simulink model "Simple_4Quad_payload_05"  (R2018b)
settings: Solver=VariableStepAuto  StartTime=0.0  StopTime=60  RelTol=1e-3
InitFcn:
  | Simple_4Quad_payload_05_const
values from neighbouring files (symbols this model uses):
  All_rho = [d1 0 0 ... (first row only)    [Colab_4Quad_model_01_const.m]    (also in Colab_4Quad_model_02_const.m; Simple_4Quad_payload_04_const.m; Simple_4Quad_payload_05_const.m; Simple_4Quad_payload_06_const.m)
  B_ob = [zeros(3);eye(3)]    [Simple_4Quad_payload_04_const.m]    (also in Simple_4Quad_payload_05_const.m; Simple_4Quad_payload_06_const.m; Simple_4Quad_payload_07_const.m; Simple_4Quad_payload_08_const.m)
  BBT_inv = ((B'*B)^(-1))*B'    [Simple_2Quad_payload_03_const.m]    (also in Simple_4Quad_payload_04_const.m = ((BR'*BR)^(-1))*BR'; Simple_4Quad_payload_05_const.m = ((BR'*BR)^(-1))*BR'; Simple_4Quad_payload_06_const.m = ((BR'*BR)^(-1))*BR'; Simple_4Quad_payload_07_const.m = ((BR'*BR)^(-1))*BR')
  BR = 1e0*eye(n)    [Simple_4Quad_payload_04_const.m]    (also in Simple_4Quad_payload_05_const.m; Simple_4Quad_payload_06_const.m; Simple_4Quad_payload_07_const.m; Simple_4Quad_payload_08_const.m)
  C_ob = [eye(3) zeros(3)]    [Simple_4Quad_payload_04_const.m]    (also in Simple_4Quad_payload_05_const.m; Simple_4Quad_payload_06_const.m; Simple_4Quad_payload_07_const.m; Simple_4Quad_payload_08_const.m)
  d1 = 0.25    [Colab_4Quad_model_01_const.m]    (also in Colab_4Quad_model_02_const.m = 0.5; Simple_4Quad_payload_01_const.m = 1; Simple_4Quad_payload_02_const.m = 1; Simple_4Quad_payload_03_const.m = 1)
  d2 = 0.25    [Colab_4Quad_model_01_const.m]    (also in Colab_4Quad_model_02_const.m = 0.5; Simple_4Quad_payload_01_const.m = 1; Simple_4Quad_payload_02_const.m = 1; Simple_4Quad_payload_03_const.m = 1)
  Des_rel_dist = 2    [Simple_4Quad_payload_01_const.m]    (also in Simple_4Quad_payload_02_const.m = 4; Simple_4Quad_payload_03_const.m = 4; Simple_4Quad_payload_04_const.m; Simple_4Quad_payload_05_const.m)
  g = 9.81    [Colab_4Quad_model_01_const.m]    (also in Colab_4Quad_model_02_const.m; Simple_2Quad_payload_01_const.m; Simple_2Quad_payload_02_const.m; Simple_2Quad_payload_03_const.m)
  gamma_0 = 1e-0*diag([1e-3;1e-0])    [Simple_2Quad_payload_03_const.m]    (also in Simple_4Quad_payload_04_const.m = 1e-0*diag([1e-6*ones(3,1);1e-0*ones(3,1)]); Simple_4Quad_payload_05_const.m = 1e-1*diag([1e-6*ones(3,1);1e-0*ones(3,1)]); Simple_4Quad_payload_06_const.m = 1e-0*diag([1e-6*ones(3,1);1e-0*ones(3,1)]); Simple_4Quad_payload_07_const.m = 1e-0*diag([1e-6*ones(3,1);1e-0*ones(3,1)]))
  gamma_1 = 1e+2*diag([1e-3;1e-0])    [Simple_2Quad_payload_03_const.m]    (also in Simple_4Quad_payload_04_const.m = 1e+2*diag([1e-6*ones(3,1);1e-0*ones(3,1)]); Simple_4Quad_payload_05_const.m = 1e+2*diag([1e-6*ones(3,1);1e-0*ones(3,1)]); Simple_4Quad_payload_06_const.m = 1e+3*diag([1e-6*ones(3,1);1e-0*ones(3,1)]); Simple_4Quad_payload_07_const.m = 1e+3*diag([1e-6*ones(3,1);1e-0*ones(3,1)]))
  Ix = 0.166667    [Colab_4Quad_model_01_const.m]    (also in Colab_4Quad_model_02_const.m = 0.02; Simple_4Quad_payload_01_const.m = 1; Simple_4Quad_payload_02_const.m = 1; Simple_4Quad_payload_03_const.m = 1)
  Iy = 0.166667    [Colab_4Quad_model_01_const.m]    (also in Colab_4Quad_model_02_const.m = 0.02; Simple_4Quad_payload_01_const.m = 1; Simple_4Quad_payload_02_const.m = 1; Simple_4Quad_payload_03_const.m = 1)
  Iz = 0.166667    [Colab_4Quad_model_01_const.m]    (also in Colab_4Quad_model_02_const.m = 0.02; Simple_4Quad_payload_01_const.m = 1; Simple_4Quad_payload_02_const.m = 1; Simple_4Quad_payload_03_const.m = 1)
  Jo = diag([Ix;Iy;Iz])    [Colab_4Quad_model_01_const.m]    (also in Colab_4Quad_model_02_const.m; Simple_4Quad_payload_04_const.m; Simple_4Quad_payload_05_const.m; Simple_4Quad_payload_06_const.m)
  Jq = diag([0.0291 0.0291 0.0552])    [Colab_4Quad_model_01_const.m]    (also in Colab_4Quad_model_02_const.m = diag([0.03 0.03 0.06]); Simple_4Quad_payload_03_const.m = 1.2416e-3 * diag([1 1 2]); Simple_4Quad_payload_04_const.m = 1 * diag([1 1 2]); Simple_4Quad_payload_05_const.m = 1 * diag([1 1 2]))
  k1 = 1    [Simple_2Quad_payload_03_const.m]    (also in Simple_4Quad_payload_04_const.m; Simple_4Quad_payload_05_const.m; Simple_4Quad_payload_06_const.m; Simple_4Quad_payload_07_const.m)
  k2 = 0.1    [Simple_2Quad_payload_03_const.m]    (also in Simple_4Quad_payload_04_const.m; Simple_4Quad_payload_05_const.m; Simple_4Quad_payload_06_const.m; Simple_4Quad_payload_07_const.m)
  ki1_N = 0    [Simple_4Quad_payload_02_const.m]    (also in Simple_4Quad_payload_03_const.m; Simple_4Quad_payload_04_const.m; Simple_4Quad_payload_05_const.m; Simple_4Quad_payload_06_const.m)
  ki2_N = 0    [Simple_4Quad_payload_02_const.m]    (also in Simple_4Quad_payload_03_const.m; Simple_4Quad_payload_04_const.m; Simple_4Quad_payload_05_const.m; Simple_4Quad_payload_06_const.m = 10)
  kp1_N = 10    [Simple_4Quad_payload_02_const.m]    (also in Simple_4Quad_payload_03_const.m; Simple_4Quad_payload_04_const.m; Simple_4Quad_payload_05_const.m = 1; Simple_4Quad_payload_06_const.m = 1)
  kp2_N = 100    [Simple_4Quad_payload_02_const.m]    (also in Simple_4Quad_payload_03_const.m; Simple_4Quad_payload_04_const.m; Simple_4Quad_payload_05_const.m = 1; Simple_4Quad_payload_06_const.m = 1)
  l = 3.1819    [Colab_4Quad_model_01_const.m]    (also in Colab_4Quad_model_02_const.m = 3; Simple_2Quad_payload_04_const.m = 1; Simple_4Quad_payload_01_const.m = 1; Simple_4Quad_payload_02_const.m = 2)
  m = 1.5    [Colab_4Quad_model_01_const.m]    (also in Colab_4Quad_model_02_const.m; Simple_2Quad_payload_04_const.m = 1; Simple_4Quad_payload_01_const.m = 1; Simple_4Quad_payload_02_const.m = 1)
  M = 1.0    (= 1)    [Colab_4Quad_model_01_const.m]    (also in Colab_4Quad_model_02_const.m; Simple_2Quad_payload_01_const.m; Simple_2Quad_payload_02_const.m; Simple_2Quad_payload_03_const.m)
  Md = 1*[1;1;1]    [Simple_2Quad_payload_04_const.m]    (also in Simple_4Quad_payload_01_const.m = 1*[1;1;1;1;1;1]; Simple_4Quad_payload_02_const.m = 1*[1;1;1;1;1;1]; Simple_4Quad_payload_03_const.m = 1*[1;1;1;1;1;1]; Simple_4Quad_payload_04_const.m = 1*[1;1;1;1;1;1])
  n = 2    [Simple_2Quad_payload_03_const.m]    (also in Simple_4Quad_payload_03_const.m = 6; Simple_4Quad_payload_04_const.m = 6; Simple_4Quad_payload_05_const.m = 6; Simple_4Quad_payload_06_const.m = 6)
  Q_ob = var_u_ob * eye(6)    [Simple_4Quad_payload_04_const.m]    (also in Simple_4Quad_payload_05_const.m; Simple_4Quad_payload_06_const.m; Simple_4Quad_payload_07_const.m; Simple_4Quad_payload_08_const.m)
  QR = 1e-0*eye(n)    [Simple_4Quad_payload_04_const.m]    (also in Simple_4Quad_payload_05_const.m = 1e-1*eye(n); Simple_4Quad_payload_06_const.m; Simple_4Quad_payload_07_const.m; Simple_4Quad_payload_08_const.m)
  R = 1e+0*eye(n)    [Simple_2Quad_payload_03_const.m]    (also in Simple_4Quad_payload_04_const.m = 1e+0*eye(m); Simple_4Quad_payload_05_const.m = 1e+0*eye(m); Simple_4Quad_payload_06_const.m; Simple_4Quad_payload_07_const.m)
  R_ob = var_y_ob * eye(3)    [Simple_4Quad_payload_04_const.m]    (also in Simple_4Quad_payload_05_const.m; Simple_4Quad_payload_06_const.m; Simple_4Quad_payload_07_const.m; Simple_4Quad_payload_08_const.m)
  rho_0 = 1e-0    (= 1)    [Simple_2Quad_payload_03_const.m]    (also in Simple_4Quad_payload_04_const.m; Simple_4Quad_payload_05_const.m = 0.1; Simple_4Quad_payload_06_const.m; Simple_4Quad_payload_07_const.m)
  rho_1 = 1e-0    (= 1)    [Simple_2Quad_payload_03_const.m]    (also in Simple_4Quad_payload_04_const.m; Simple_4Quad_payload_05_const.m; Simple_4Quad_payload_06_const.m; Simple_4Quad_payload_07_const.m)
libraries: simulink x8
(part 3 of 3)

== matlab function Simple_4Quad_payload_05/Dynamic model of the entire system/Dynamic Model  ==
  data: DD_PHI output; D_PHI output; D_Omegao output; D_omegai_1 output; D_omegai_2 output; D_omegai_3 output; D_omegai_4 output; D_Omega_Q1 output; D_Omega_Q2 output; D_Omega_Q3 output; D_Omega_Q4 output; Dq1 output; Dq2 output; Dq3 output; Dq4 output; DDq1 output; DDq2 output; DDq3 output; DDq4 output; PHI input; Omegao input; omegai1 input; omegai2 input; omegai3 input; omegai4 input; Omega_q1 input; Omega_q2 input; Omega_q3 input; Omega_q4 input; q1 input; q2 input; q3 input; q4 input; DD_Po output; M parameter; Jo parameter; g parameter; m parameter; l parameter; Tau_q1 input; Tau_q2 input; Tau_q3 input; Tau_q4 input; Jq parameter; U1_local input; U2_local input; U3_local input; U4_local input; All_rho parameter
function [DD_PHI,D_PHI,D_Omegao,D_omegai_1,D_omegai_2,D_omegai_3,D_omegai_4,D_Omega_Q1,D_Omega_Q2,D_Omega_Q3,D_Omega_Q4,Dq1,Dq2,Dq3,Dq4,DDq1,DDq2,DDq3,DDq4,DD_Po] = ...
    fcn(PHI,Omegao,omegai1,omegai2,omegai3,omegai4,Omega_q1,Omega_q2,Omega_q3,Omega_q4,q1,q2,q3,q4,M,Jo,g,m, l,Tau_q1,Tau_q2,Tau_q3,Tau_q4, Jq, U1_local,U2_local,U3_local,U4_local, All_rho)

phi = PHI(1);
theta = PHI(2);
psi = PHI(3);

Ro = [cos(psi)*cos(theta) cos(psi)*sin(theta)*sin(phi)-sin(psi)*cos(phi) cos(psi)*sin(theta)*cos(phi)+sin(psi)*sin(phi);
    sin(psi)*cos(theta) sin(psi)*sin(theta)*sin(phi)+cos(psi)*cos(phi) sin(psi)*sin(theta)*cos(phi)-cos(psi)*sin(phi);
    -sin(theta) cos(theta)*sin(phi) cos(theta)*cos(phi)];

r1 = All_rho(1,:)';
r2 = All_rho(2,:)';
r3 = All_rho(3,:)';
r4 = All_rho(4,:)';

G = [0;0;-g];

%% 
Ui_local = struct('val',repmat({zeros(3,1)},4,1));
ri = struct('val',repmat({zeros(3,1)},4,1));
ri_skew = struct('val',repmat({zeros(3)},4,1));
qi_body = struct('val',repmat({zeros(3,1)},4,1));
qi_inert = struct('val',repmat({zeros(3,1)},4,1));
qi_inert_skew = struct('val',repmat({zeros(3)},4,1));
Mq = struct('val',repmat({zeros(3,1)},4,1));
Omega_Qi_skew = struct('val',repmat({zeros(3)},4,1));
Omega_Qi = struct('val',repmat({zeros(3,1)},4,1));
D_Omega_Qi = struct('val',repmat({zeros(3,1)},4,1));

Ui_local(1).val = U1_local;
Ui_local(2).val = U2_local;
Ui_local(3).val = U3_local;
Ui_local(4).val = U4_local;

ri(1).val = r1;
ri(2).val = r2;
ri(3).val = r3;
ri(4).val = r4;

ri_skew(1).val = ... 
    [0 -r1(3) r1(2);
    r1(3) 0 -r1(1);
    -r1(2) r1(1) 0];

ri_skew(2).val = ... 
    [0 -r2(3) r2(2);
    r2(3) 0 -r2(1);
    -r2(2) r2(1) 0];

ri_skew(3).val = ... 
    [0 -r3(3) r3(2);
    r3(3) 0 -r3(1);
    -r3(2) r3(1) 0];

ri_skew(4).val = ... 
    [0 -r4(3) r4(2);
    r4(3) 0 -r4(1);
    -r4(2) r4(1) 0];

qi_body(1).val = q1;
qi_body(2).val = q2;
qi_body(3).val = q3;
qi_body(4).val = q4;

qi_inert(1).val = Ro * qi_body(1).val;
qi_inert(2).val = Ro * qi_body(2).val;
qi_inert(3).val = Ro * qi_body(3).val;
qi_inert(4).val = Ro * qi_body(4).val;

qi_inert_skew(1).val = ...
    [0 -qi_inert(1).val(3) qi_inert(1).val(2);
    qi_inert(1).val(3) 0 -qi_inert(1).val(1);
    -qi_inert(1).val(2) qi_inert(1).val(1) 0];

qi_inert_skew(2).val = ...
    [0 -qi_inert(2).val(3) qi_inert(2).val(2);
    qi_inert(2).val(3) 0 -qi_inert(2).val(1);
    -qi_inert(2).val(2) qi_inert(2).val(1) 0];

qi_inert_skew(3).val = ...
    [0 -qi_inert(3).val(3) qi_inert(3).val(2);
    qi_inert(3).val(3) 0 -qi_inert(3).val(1);
    -qi_inert(3).val(2) qi_inert(3).val(1) 0];

qi_inert_skew(4).val = ...
    [0 -qi_inert(4).val(3) qi_inert(4).val(2);
    qi_inert(4).val(3) 0 -qi_inert(4).val(1);
    -qi_inert(4).val(2) qi_inert(4).val(1) 0];

Omegao_skew = ...
    [0 -Omegao(3) Omegao(2);
    Omegao(3) 0 -Omegao(1);
    -Omegao(2) Omegao(1) 0];

Mag2_omegai = ...
    [omegai1'*omegai1;
    omegai2'*omegai2;
    omegai3'*omegai3;
    omegai4'*omegai4];

Mq(1).val = Tau_q1;
Mq(2).val = Tau_q2;
Mq(3).val = Tau_q3;
Mq(4).val = Tau_q4;

Omega_Qi(1).val = Omega_q1;
Omega_Qi(2).val = Omega_q2;
Omega_Qi(3).val = Omega_q3;
Omega_Qi(4).val = Omega_q4;

Omega_Qi_skew(1).val = ...
    [0 -Omega_Qi(1).val(3) Omega_Qi(1).val(2);
    Omega_Qi(1).val(3) 0 -Omega_Qi(1).val(1);
    -Omega_Qi(1).val(2) Omega_Qi(1).val(1) 0];

Omega_Qi_skew(2).val = ...
    [0 -Omega_Qi(2).val(3) Omega_Qi(2).val(2);
    Omega_Qi(2).val(3) 0 -Omega_Qi(2).val(1);
    -Omega_Qi(2).val(2) Omega_Qi(2).val(1) 0];

Omega_Qi_skew(3).val = ...
    [0 -Omega_Qi(3).val(3) Omega_Qi(3).val(2);
    Omega_Qi(3).val(3) 0 -Omega_Qi(3).val(1);
    -Omega_Qi(3).val(2) Omega_Qi(3).val(1) 0];

Omega_Qi_skew(4).val = ...
    [0 -Omega_Qi(4).val(3) Omega_Qi(4).val(2);
    Omega_Qi(4).val(3) 0 -Omega_Qi(4).val(1);
    -Omega_Qi(4).val(2) Omega_Qi(4).val(1) 0];


%% Dynamics of the entire system
u_DDP = zeros(3,1);
u_DOmega = zeros(3,1);
term_g_DDP = (M*G);
term_DOmega_DDP = zeros(3);
term_Omega2_DDP = zeros(3,1);
term_omegai2_DDP = zeros(3,1);
term_DOmega_DOmega = zeros(3);
term_Omega2_DOmega = zeros(3,1);
term_DDP_DOmega = zeros(3);
term_omegai2_DOmega = zeros(3,1);
term_g_DOmega = zeros(3,1);

M_tot = zeros(18,18);
F_tot = zeros(18,1);

for i=1:4
    u_DDP = u_DDP + ( Ro * Ui_local(i).val );
    u_DOmega = u_DOmega + ( ri_skew(i).val * Ui_local(i).val );
    term_DOmega_DDP = term_DOmega_DDP + ( m * qi_inert(i).val * qi_inert(i).val' * Ro * ri_skew(i).val );
    term_Omega2_DDP = term_Omega2_DDP + ( m * qi_inert(i).val * qi_inert(i).val' * Ro * Omegao_skew * Omegao_skew * ri(i).val );
    term_omegai2_DDP = term_omegai2_DDP + ( m * l * Mag2_omegai(i) * qi_inert(i).val );
    term_DOmega_DOmega = term_DOmega_DOmega + ( m * ri_skew(i).val * Ro' * qi_inert(i).val * qi_inert(i).val' * Ro * ri_skew(i).val );
    term_Omega2_DOmega = term_Omega2_DOmega + ( m * ri_skew(i).val * Ro' * qi_inert(i).val * qi_inert(i).val' * Ro * Omegao_skew * Omegao_skew * ri(i).val );
    term_omegai2_DOmega = term_omegai2_DOmega + ( m * l * ri_skew(i).val * Ro' * Mag2_omegai(i) * qi_inert(i).val );
    term_DDP_DOmega = term_DDP_DOmega + ( m * ri_skew(i).val * Ro' * qi_inert(i).val * qi_inert(i).val' );
    term_g_DOmega = term_g_DOmega + ( m * ri_skew(i).val * Ro' * qi_inert(i).val * qi_inert(i).val' * G );
    
    M_tot(6+(i-1)*3+1:6+(i-1)*3+3,1:3) = -1 * m * qi_inert_skew(i).val;
    M_tot(6+(i-1)*3+1:6+(i-1)*3+3,4:6) = m * qi_inert_skew(i).val * Ro * ri_skew(i).val;
    M_tot(6+(i-1)*3+1:6+(i-1)*3+3,6+(i-1)*3+1:6+(i-1)*3+3) = m * l * eye(3);
    
    F_tot(6+(i-1)*3+1:6+(i-1)*3+3,1) = ( m * qi_inert_skew(i).val * G ) + ( m * qi_inert_skew(i).val * Ro * Omegao_skew * Omegao_skew * ri(i).val ) - ...
        ( qi_inert_skew(i).val * Ui_local(i).val ); 
    
    D_Omega_Qi(i).val = (Jq ^ (-1)) * ( Mq(i).val - (Omega_Qi_skew(i).val * Jq * Omega_Qi(i).val) );
end

M_tot(1:3,1:3) = M * eye(3);
M_tot(1:3,4:6) = -1 * term_DOmega_DDP;

M_tot(4:6,1:3) = term_DDP_DOmega;
M_tot(4:6,4:6) = Jo - term_DOmega_DOmega;

F_tot(1:3,1) = u_DDP + term_g_DDP - term_omegai2_DDP - term_Omega2_DDP;
F_tot(4:6,1) = u_DOmega - term_g_DOmega - (Omegao_skew * Jo * Omegao) - term_omegai2_DOmega - term_Omega2_DOmega;

DX_tot = M_tot^(-1) * F_tot;

DD_Po = DX_tot(1:3,1);
D_Omegao = DX_tot(4:6,1);
D_omegai_1 = DX_tot(7:9,1);
D_omegai_2 = DX_tot(10:12,1);
D_omegai_3 = DX_tot(13:15,1);
D_omegai_4 = DX_tot(16:18,1);

D_Omega_Q1 = D_Omega_Qi(1).val;
D_Omega_Q2 = D_Omega_Qi(2).val;
D_Omega_Q3 = D_Omega_Qi(3).val;
D_Omega_Q4 = D_Omega_Qi(4).val;

%% Angles of links and their rates
omega1_skew = ...
    [0 -omegai1(3) omegai1(2);
    omegai1(3) 0 -omegai1(1);
    -omegai1(2) omegai1(1) 0];

omega2_skew = ...
    [0 -omegai2(3) omegai2(2);
    omegai2(3) 0 -omegai2(1);
    -omegai2(2) omegai2(1) 0];

omega3_skew = ...
    [0 -omegai3(3) omegai3(2);
    omegai3(3) 0 -omegai3(1);
    -omegai3(2) omegai3(1) 0];

omega4_skew = ...
    [0 -omegai4(3) omegai4(2);
    omegai4(3) 0 -omegai4(1);
    -omegai4(2) omegai4(1) 0];

Dq1 = omega1_skew * q1;
Dq2 = omega2_skew * q2;
Dq3 = omega3_skew * q3;
Dq4 = omega4_skew * q4;

Domega1_skew = ...
    [0 -D_omegai_1(3) D_omegai_1(2);
    D_omegai_1(3) 0 -D_omegai_1(1);
    -D_omegai_1(2) D_omegai_1(1) 0];

Domega2_skew = ...
    [0 -D_omegai_2(3) D_omegai_2(2);
    D_omegai_2(3) 0 -D_omegai_2(1);
    -D_omegai_2(2) D_omegai_2(1) 0];

Domega3_skew = ...
    [0 -D_omegai_3(3) D_omegai_3(2);
    D_omegai_3(3) 0 -D_omegai_3(1);
    -D_omegai_3(2) D_omegai_3(1) 0];

Domega4_skew = ...
    [0 -D_omegai_4(3) D_omegai_4(2);
    D_omegai_4(3) 0 -D_omegai_4(1);
    -D_omegai_4(2) D_omegai_4(1) 0];

DDq1 = Domega1_skew*q1 + omega1_skew*Dq1;
DDq2 = Domega2_skew*q2 + omega2_skew*Dq2;
DDq3 = Domega3_skew*q3 + omega3_skew*Dq3;
DDq4 = Domega4_skew*q4 + omega4_skew*Dq4;

%% Euler angles of the payload and their rates
R_f_o = [1 0 -sin(theta);
    0 cos(phi) cos(theta)*sin(phi);
    0 -sin(phi) cos(theta)*cos(phi)];

D_PHI = (R_f_o^-1) * Omegao;

DR_f_o = [0 0 -D_PHI(2)*cos(theta);
    0 -D_PHI(1)*sin(phi) (-D_PHI(2)*sin(theta)*sin(phi))+(D_PHI(1)*cos(theta)*cos(phi));
    0 -D_PHI(1)*cos(phi) (-D_PHI(2)*sin(theta)*cos(phi))-(D_PHI(1)*cos(theta)*sin(phi))];

DD_PHI = (R_f_o^-1) * ( D_Omegao - DR_f_o*D_PHI );

end

== matlab function Simple_4Quad_payload_05/Controllers and Observers/Controller and Observer - Agent2/Controller Interpreter #2 ==
  data: ut_2 input; PHI_d_2 output
function PHI_d_2 = fcn(ut_2)

%%
fT_2 = sqrt((ut_2(1)^2)+(ut_2(2)^2)+(ut_2(3)^2));
psi_d_2 = 0;
phi_d_2 = asin( min(max(((sin(psi_d_2)*ut_2(1) - cos(psi_d_2)*ut_2(2)) / (fT_2+1e-3)),-1),1) );
theta_d_2 = atan( (cos(psi_d_2)*ut_2(1) + sin(psi_d_2)*ut_2(2)) / (ut_2(3)+1e-3) );
PHI_d_2 = [phi_d_2;theta_d_2;psi_d_2]; 

end

== matlab function Simple_4Quad_payload_05/Controllers and Observers/Controlelr and Observer - Agent3/Controller Interpreter #3 ==
  data: ut_3 input; PHI_d_3 output
function PHI_d_3 = fcn(ut_3)

%%
fT_3 = sqrt((ut_3(1)^2)+(ut_3(2)^2)+(ut_3(3)^2));
psi_d_3 = 0;
phi_d_3 = asin( min(max(((sin(psi_d_3)*ut_3(1) - cos(psi_d_3)*ut_3(2)) / (fT_3+1e-3)),-1),1) );
theta_d_3 = atan( (cos(psi_d_3)*ut_3(1) + sin(psi_d_3)*ut_3(2)) / (ut_3(3)+1e-3) );
PHI_d_3 = [phi_d_3;theta_d_3;psi_d_3]; 

end

== matlab function Simple_4Quad_payload_05/Controllers and Observers/Controller and Observer - Agent2/Rotational #2/CARE ==
  data: P input; a_hat input; BR parameter; R parameter; DP output; QR parameter
function DP = fcn(P,a_hat,BR,R,QR)

DP = a_hat*P + P*a_hat' - P*BR*R*BR'*P + 2*QR;

end

== matlab function Simple_4Quad_payload_05/Controllers and Observers/Controller and Observer - Agent2/Rotational #2/Differentiator/Sliding differentiator ==
  data: u output; u1 input; e input; n parameter; k1 parameter
function u = fcn(u1,e,n,k1)

b=k1;

ABS = zeros(n,1);
for i=1:n
    if e(i)>0
        ABS(i) = e(i);
    else
        ABS(i) = -e(i);
    end
end
SGN = e ./ (ABS + 0.01);

u = u1 - b*(ABS.^0.5).*SGN;

end

== matlab function Simple_4Quad_payload_05/Controllers and Observers/Controller and Observer - Agent2/Rotation_Q2/D Phi ==
  data: Omega_Q2 input; D_PHI_Q2 output; PHI_Q2 input
function D_PHI_Q2 = fcn(Omega_Q2,PHI_Q2)

phi_q2 = PHI_Q2(1);
theta_q2 = PHI_Q2(2);

Rm_Q2 = [1 0 -sin(theta_q2);
    0 cos(phi_q2) cos(theta_q2)*sin(phi_q2);
    0 -sin(phi_q2) cos(theta_q2)*cos(phi_q2)];

D_PHI_Q2 = (Rm_Q2)^(-1) * Omega_Q2;


end

== matlab function Simple_4Quad_payload_05/Controllers and Observers/Controller and Observer - Agent2/Rotational #2/Differentiator/Sliding differentiator1 ==
  data: Du1 output; e input; n parameter; k2 parameter
function Du1 = fcn(e,n,k2)

a=k2;

ABS = zeros(n,1);
for i=1:n
    if e(i)>0
        ABS(i) = e(i);
    else
        ABS(i) = -e(i);
    end
end
SGN = e ./ (ABS + 0.01);

Du1 = - a*SGN;

end

== matlab function Simple_4Quad_payload_05/Controllers and Observers/Controller and Observer - Agent2/Rotational #2/g-Estimator ==
  data: sigma input; g_hat input; P input; rho_1 parameter; gamma_1 parameter; Dg_hat output
function Dg_hat = fcn(sigma,g_hat,P,rho_1,gamma_1)

Dg_hat = - gamma_1 * P * sigma - rho_1 * gamma_1 * g_hat;

end

== matlab function Simple_4Quad_payload_05/Controllers and Observers/Controller and Observer - Agent2/Rotational #2/g-Estimator1 ==
  data: sigma input; x input; P input; rho_0 parameter; gamma_0 parameter; Da_hat output; a_hat input
function Da_hat = fcn(sigma,x,P,rho_0,gamma_0,a_hat)

DVa_hat = - gamma_0 * P * diag(sigma) * (x - sigma) - rho_0 * gamma_0 * diag(a_hat);

Da_hat = diag(DVa_hat);

end

== matlab function Simple_4Quad_payload_05/Controllers and Observers/Controller and Observer - Agent2/Rotational #2/main ==
  data: sigma input; zeta input; u output; Dy_d input; R parameter; P input; a_hat input; BR parameter; g_hat input; x input; QR parameter; BBT_inv parameter; n parameter
function u = fcn(sigma,zeta,Dy_d,R,P,a_hat,BR,g_hat,x,QR,BBT_inv,n)

u1 = (1/2) * R * BR' * P * sigma;
u2 = BBT_inv * (Dy_d - a_hat*x + (eye(n) + 2*(((P)^(-1)*QR)) + a_hat)*sigma - g_hat - zeta) - (3/4) * R * BR' * P * sigma;

u = u1 + u2;

end

== matlab function Simple_4Quad_payload_05/Controllers and Observers/Controller and Observer - Agent2/Rotational #2/variable change ==
  data: X input; Xd input; x_mod output; u input; xd_mod output; e_mod output
function [x_mod,xd_mod,e_mod] = fcn(X,Xd,u)

x_mod = X;

xd_mod = [Xd;u(1:3)];

e_mod = xd_mod - x_mod;


end

== matlab function Simple_4Quad_payload_05/Controllers and Observers/Controlelr and Observer - Agent3/Rotation_Q3/D Phi ==
  data: Omega_Q3 input; D_PHI_Q3 output; PHI_Q3 input
function D_PHI_Q3 = fcn(Omega_Q3,PHI_Q3)

phi_q3 = PHI_Q3(1);
theta_q3 = PHI_Q3(2);

Rm_Q3 = [1 0 -sin(theta_q3);
    0 cos(phi_q3) cos(theta_q3)*sin(phi_q3);
    0 -sin(phi_q3) cos(theta_q3)*cos(phi_q3)];

D_PHI_Q3 = (Rm_Q3)^(-1) * Omega_Q3;


end

== matlab function Simple_4Quad_payload_05/Controllers and Observers/Controller and Observer - Agent4/Rotation_Q4/D Phi ==
  data: Omega_Q4 input; D_PHI_Q4 output; PHI_Q4 input
function D_PHI_Q4 = fcn(Omega_Q4,PHI_Q4)

phi_q4 = PHI_Q4(1);
theta_q4 = PHI_Q4(2);

Rm_Q4 = [1 0 -sin(theta_q4);
    0 cos(phi_q4) cos(theta_q4)*sin(phi_q4);
    0 -sin(phi_q4) cos(theta_q4)*cos(phi_q4)];

D_PHI_Q4 = (Rm_Q4)^(-1) * Omega_Q4;


end

== matlab function Simple_4Quad_payload_05/Controllers and Observers/MATLAB Function ==
  data: q_des input; q1_des output; q2_des output; q3_des output; q4_des output
function [q1_des,q2_des,q3_des,q4_des] = fcn(q_des)

q1_des = q_des(:,1);
q2_des = q_des(:,2);
q3_des = q_des(:,3);
q4_des = q_des(:,4);

end

== matlab function Simple_4Quad_payload_05/Controllers and Observers/Controlelr and Observer - Agent3/Rotational #3/CARE ==
  data: P input; a_hat input; BR parameter; R parameter; DP output; QR parameter
function DP = fcn(P,a_hat,BR,R,QR)

DP = a_hat*P + P*a_hat' - P*BR*R*BR'*P + 2*QR;

end

== matlab function Simple_4Quad_payload_05/Controllers and Observers/Controlelr and Observer - Agent3/Rotational #3/Differentiator/Sliding differentiator ==
  data: u output; u1 input; e input; n parameter; k1 parameter
function u = fcn(u1,e,n,k1)

b=k1;

ABS = zeros(n,1);
for i=1:n
    if e(i)>0
        ABS(i) = e(i);
    else
        ABS(i) = -e(i);
    end
end
SGN = e ./ (ABS + 0.01);

u = u1 - b*(ABS.^0.5).*SGN;

end

== matlab function Simple_4Quad_payload_05/Controllers and Observers/Controlelr and Observer - Agent3/Rotational #3/Differentiator/Sliding differentiator1 ==
  data: Du1 output; e input; n parameter; k2 parameter
function Du1 = fcn(e,n,k2)

a=k2;

ABS = zeros(n,1);
for i=1:n
    if e(i)>0
        ABS(i) = e(i);
    else
        ABS(i) = -e(i);
    end
end
SGN = e ./ (ABS + 0.01);

Du1 = - a*SGN;

end

== matlab function Simple_4Quad_payload_05/Controllers and Observers/Controlelr and Observer - Agent3/Rotational #3/g-Estimator ==
  data: sigma input; g_hat input; P input; rho_1 parameter; gamma_1 parameter; Dg_hat output
function Dg_hat = fcn(sigma,g_hat,P,rho_1,gamma_1)

Dg_hat = - gamma_1 * P * sigma - rho_1 * gamma_1 * g_hat;

end

== matlab function Simple_4Quad_payload_05/Controllers and Observers/Controlelr and Observer - Agent3/Rotational #3/g-Estimator1 ==
  data: sigma input; x input; P input; rho_0 parameter; gamma_0 parameter; Da_hat output; a_hat input
function Da_hat = fcn(sigma,x,P,rho_0,gamma_0,a_hat)

DVa_hat = - gamma_0 * P * diag(sigma) * (x - sigma) - rho_0 * gamma_0 * diag(a_hat);

Da_hat = diag(DVa_hat);

end

== matlab function Simple_4Quad_payload_05/Controllers and Observers/Controlelr and Observer - Agent3/Rotational #3/main ==
  data: sigma input; zeta input; u output; Dy_d input; R parameter; P input; a_hat input; BR parameter; g_hat input; x input; QR parameter; BBT_inv parameter; n parameter
function u = fcn(sigma,zeta,Dy_d,R,P,a_hat,BR,g_hat,x,QR,BBT_inv,n)

u1 = (1/2) * R * BR' * P * sigma;
u2 = BBT_inv * (Dy_d - a_hat*x + (eye(n) + 2*(((P)^(-1)*QR)) + a_hat)*sigma - g_hat - zeta) - (3/4) * R * BR' * P * sigma;

u = u1 + u2;

end

== matlab function Simple_4Quad_payload_05/Controllers and Observers/Controlelr and Observer - Agent3/Rotational #3/variable change ==
  data: X input; Xd input; x_mod output; u input; xd_mod output; e_mod output
function [x_mod,xd_mod,e_mod] = fcn(X,Xd,u)

x_mod = X;

xd_mod = [Xd;u(1:3)];

e_mod = xd_mod - x_mod;


end

== matlab function Simple_4Quad_payload_05/Controllers and Observers/Cotnroller and Observer - Agent1 /Observer1/Kalman_Filter1 ==
  data: P_ob input; DP_ob output; xhat_ob input; Dxhat_ob output; Q_ob parameter; R_ob parameter; C_ob parameter; B_ob parameter; wo input; Dwo input; Rel_Posi_local input; Rel_Acci_local input; Agent_Num input; All_rho parameter
function [DP_ob,Dxhat_ob] = fcn(P_ob,xhat_ob,Q_ob, R_ob, C_ob, B_ob,wo,Dwo,Rel_Posi_local,Rel_Acci_local,Agent_Num,All_rho)

rhoi = All_rho(Agent_Num,:)';

wo_skew = [...
    0 -wo(3) wo(2);
    wo(3) 0 -wo(1);
    -wo(2) wo(1) 0];

Dwo_skew = [...
    0 -Dwo(3) Dwo(2);
    Dwo(3) 0 -Dwo(1);
    -Dwo(2) Dwo(1) 0];

A1_ob = wo_skew * wo_skew + Dwo_skew;
A2_ob = 2*wo_skew;

A_ob = [zeros(3) eye(3);
    -A1_ob -A2_ob];

y_ob = Rel_Posi_local - rhoi;
u_ob = Rel_Acci_local - A1_ob*rhoi;

DP_ob = A_ob'*P_ob + P_ob*A_ob - P_ob*C_ob'*R_ob*C_ob*P_ob + Q_ob;
K_ob = P_ob * C_ob' * R_ob;
Dxhat_ob = A_ob*xhat_ob + B_ob*u_ob + K_ob*(y_ob - C_ob*xhat_ob);

end

== matlab function Simple_4Quad_payload_05/Controllers and Observers/Cotnroller and Observer - Agent1 /Observer1/Observer_Finalization1 ==
  data: xhati input; qhati output; Dqhati output
function [qhati,Dqhati] = fcn(xhati)

qhati = xhati(1:3);
Dqhati = xhati(4:6);

end

== matlab function Simple_4Quad_payload_05/Controllers and Observers/Controller and Observer - Agent2/Observer2/Kalman_Filter2 ==
  data: P_ob input; DP_ob output; xhat_ob input; Dxhat_ob output; Q_ob parameter; R_ob parameter; C_ob parameter; B_ob parameter; wo input; Dwo input; Rel_Posi_local input; Rel_Acci_local input; Agent_Num input; All_rho parameter
function [DP_ob,Dxhat_ob] = fcn(P_ob,xhat_ob,Q_ob, R_ob, C_ob, B_ob,wo,Dwo,Rel_Posi_local,Rel_Acci_local,Agent_Num,All_rho)

rhoi = All_rho(Agent_Num,:)';

wo_skew = [...
    0 -wo(3) wo(2);
    wo(3) 0 -wo(1);
    -wo(2) wo(1) 0];

Dwo_skew = [...
    0 -Dwo(3) Dwo(2);
    Dwo(3) 0 -Dwo(1);
    -Dwo(2) Dwo(1) 0];

A1_ob = wo_skew * wo_skew + Dwo_skew;
A2_ob = 2*wo_skew;

A_ob = [zeros(3) eye(3);
    -A1_ob -A2_ob];

y_ob = Rel_Posi_local - rhoi;
u_ob = Rel_Acci_local - A1_ob*rhoi;

DP_ob = A_ob'*P_ob + P_ob*A_ob - P_ob*C_ob'*R_ob*C_ob*P_ob + Q_ob;
K_ob = P_ob * C_ob' * R_ob;
Dxhat_ob = A_ob*xhat_ob + B_ob*u_ob + K_ob*(y_ob - C_ob*xhat_ob);

end

== matlab function Simple_4Quad_payload_05/Controllers and Observers/Controller and Observer - Agent4/Controller Interpreter #4 ==
  data: ut_4 input; PHI_d_4 output
function PHI_d_4 = fcn(ut_4)

%%
fT_4 = sqrt((ut_4(1)^2)+(ut_4(2)^2)+(ut_4(3)^2));
psi_d_4 = 0;
phi_d_4 = asin( min(max(((sin(psi_d_4)*ut_4(1) - cos(psi_d_4)*ut_4(2)) / (fT_4+1e-3)),-1),1) );
theta_d_4 = atan( (cos(psi_d_4)*ut_4(1) + sin(psi_d_4)*ut_4(2)) / (ut_4(3)+1e-3) );
PHI_d_4 = [phi_d_4;theta_d_4;psi_d_4]; 

end

== matlab function Simple_4Quad_payload_05/Controllers and Observers/Controller and Observer - Agent2/Observer2/Observer_Finalization2 ==
  data: xhati input; qhati output; Dqhati output
function [qhati,Dqhati] = fcn(xhati)

qhati = xhati(1:3);
Dqhati = xhati(4:6);

end

== matlab function Simple_4Quad_payload_05/Controllers and Observers/Controller and Observer - Agent4/Rotational #4/CARE ==
  data: P input; a_hat input; BR parameter; R parameter; DP output; QR parameter
function DP = fcn(P,a_hat,BR,R,QR)

DP = a_hat*P + P*a_hat' - P*BR*R*BR'*P + 2*QR;

end

== matlab function Simple_4Quad_payload_05/Controllers and Observers/Controller and Observer - Agent4/Rotational #4/Differentiator/Sliding differentiator ==
  data: u output; u1 input; e input; n parameter; k1 parameter
function u = fcn(u1,e,n,k1)

b=k1;

ABS = zeros(n,1);
for i=1:n
    if e(i)>0
        ABS(i) = e(i);
    else
        ABS(i) = -e(i);
    end
end
SGN = e ./ (ABS + 0.01);

u = u1 - b*(ABS.^0.5).*SGN;

end

== matlab function Simple_4Quad_payload_05/Controllers and Observers/Controller and Observer - Agent4/Rotational #4/Differentiator/Sliding differentiator1 ==
  data: Du1 output; e input; n parameter; k2 parameter
function Du1 = fcn(e,n,k2)

a=k2;

ABS = zeros(n,1);
for i=1:n
    if e(i)>0
        ABS(i) = e(i);
    else
        ABS(i) = -e(i);
    end
end
SGN = e ./ (ABS + 0.01);

Du1 = - a*SGN;

end

== matlab function Simple_4Quad_payload_05/Controllers and Observers/Controller and Observer - Agent4/Rotational #4/g-Estimator ==
  data: sigma input; g_hat input; P input; rho_1 parameter; gamma_1 parameter; Dg_hat output
function Dg_hat = fcn(sigma,g_hat,P,rho_1,gamma_1)

Dg_hat = - gamma_1 * P * sigma - rho_1 * gamma_1 * g_hat;

end

== matlab function Simple_4Quad_payload_05/Controllers and Observers/Controller and Observer - Agent4/Rotational #4/g-Estimator1 ==
  data: sigma input; x input; P input; rho_0 parameter; gamma_0 parameter; Da_hat output; a_hat input
function Da_hat = fcn(sigma,x,P,rho_0,gamma_0,a_hat)

DVa_hat = - gamma_0 * P * diag(sigma) * (x - sigma) - rho_0 * gamma_0 * diag(a_hat);

Da_hat = diag(DVa_hat);

end

== matlab function Simple_4Quad_payload_05/Controllers and Observers/Controller and Observer - Agent4/Rotational #4/main ==
  data: sigma input; zeta input; u output; Dy_d input; R parameter; P input; a_hat input; BR parameter; g_hat input; x input; QR parameter; BBT_inv parameter; n parameter
function u = fcn(sigma,zeta,Dy_d,R,P,a_hat,BR,g_hat,x,QR,BBT_inv,n)

u1 = (1/2) * R * BR' * P * sigma;
u2 = BBT_inv * (Dy_d - a_hat*x + (eye(n) + 2*(((P)^(-1)*QR)) + a_hat)*sigma - g_hat - zeta) - (3/4) * R * BR' * P * sigma;

u = u1 + u2;

end

== matlab function Simple_4Quad_payload_05/Controllers and Observers/Controller and Observer - Agent4/Rotational #4/variable change ==
  data: X input; Xd input; x_mod output; u input; xd_mod output; e_mod output
function [x_mod,xd_mod,e_mod] = fcn(X,Xd,u)

x_mod = X;

xd_mod = [Xd;u(1:3)];

e_mod = xd_mod - x_mod;


end

== matlab function Simple_4Quad_payload_05/Controllers and Observers/Controlelr and Observer - Agent3/Observer3/Kalman_Filter3 ==
  data: P_ob input; DP_ob output; xhat_ob input; Dxhat_ob output; Q_ob parameter; R_ob parameter; C_ob parameter; B_ob parameter; wo input; Dwo input; Rel_Posi_local input; Rel_Acci_local input; Agent_Num input; All_rho parameter
function [DP_ob,Dxhat_ob] = fcn(P_ob,xhat_ob,Q_ob, R_ob, C_ob, B_ob,wo,Dwo,Rel_Posi_local,Rel_Acci_local,Agent_Num,All_rho)

rhoi = All_rho(Agent_Num,:)';

wo_skew = [...
    0 -wo(3) wo(2);
    wo(3) 0 -wo(1);
    -wo(2) wo(1) 0];

Dwo_skew = [...
    0 -Dwo(3) Dwo(2);
    Dwo(3) 0 -Dwo(1);
    -Dwo(2) Dwo(1) 0];

A1_ob = wo_skew * wo_skew + Dwo_skew;
A2_ob = 2*wo_skew;

A_ob = [zeros(3) eye(3);
    -A1_ob -A2_ob];

y_ob = Rel_Posi_local - rhoi;
u_ob = Rel_Acci_local - A1_ob*rhoi;

DP_ob = A_ob'*P_ob + P_ob*A_ob - P_ob*C_ob'*R_ob*C_ob*P_ob + Q_ob;
K_ob = P_ob * C_ob' * R_ob;
Dxhat_ob = A_ob*xhat_ob + B_ob*u_ob + K_ob*(y_ob - C_ob*xhat_ob);

end

== matlab function Simple_4Quad_payload_05/Controllers and Observers/Controlelr and Observer - Agent3/Observer3/Observer_Finalization3 ==
  data: xhati input; qhati output; Dqhati output
function [qhati,Dqhati] = fcn(xhati)

qhati = xhati(1:3);
Dqhati = xhati(4:6);

end

== matlab function Simple_4Quad_payload_05/Controllers and Observers/Controller and Observer - Agent4/Observer4/Kalman_Filter4 ==
  data: P_ob input; DP_ob output; xhat_ob input; Dxhat_ob output; Q_ob parameter; R_ob parameter; C_ob parameter; B_ob parameter; wo input; Dwo input; Rel_Posi_local input; Rel_Acci_local input; Agent_Num input; All_rho parameter
function [DP_ob,Dxhat_ob] = fcn(P_ob,xhat_ob,Q_ob, R_ob, C_ob, B_ob,wo,Dwo,Rel_Posi_local,Rel_Acci_local,Agent_Num,All_rho)

rhoi = All_rho(Agent_Num,:)';

wo_skew = [...
    0 -wo(3) wo(2);
    wo(3) 0 -wo(1);
    -wo(2) wo(1) 0];

Dwo_skew = [...
    0 -Dwo(3) Dwo(2);
    Dwo(3) 0 -Dwo(1);
    -Dwo(2) Dwo(1) 0];

A1_ob = wo_skew * wo_skew + Dwo_skew;
A2_ob = 2*wo_skew;

A_ob = [zeros(3) eye(3);
    -A1_ob -A2_ob];

y_ob = Rel_Posi_local - rhoi;
u_ob = Rel_Acci_local - A1_ob*rhoi;

DP_ob = A_ob'*P_ob + P_ob*A_ob - P_ob*C_ob'*R_ob*C_ob*P_ob + Q_ob;
K_ob = P_ob * C_ob' * R_ob;
Dxhat_ob = A_ob*xhat_ob + B_ob*u_ob + K_ob*(y_ob - C_ob*xhat_ob);

end

== matlab function Simple_4Quad_payload_05/Controllers and Observers/Controller and Observer - Agent4/Observer4/Observer_Finalization4 ==
  data: xhati input; qhati output; Dqhati output
function [qhati,Dqhati] = fcn(xhati)

qhati = xhati(1:3);
Dqhati = xhati(4:6);

end

== matlab function Simple_4Quad_payload_05/Relative measurements/Relative position measurements in payload local frame ==
  data: PHI input; Rel_Pos_local1 output; ro input; r1 input; r2 input; r3 input; r4 input; Rel_Pos_local2 output; Rel_Pos_local3 output; Rel_Pos_local4 output
function [Rel_Pos_local1,Rel_Pos_local2,Rel_Pos_local3,Rel_Pos_local4] = fcn(PHI,ro,r1,r2,r3,r4)

phi = PHI(1);
theta = PHI(2);
psi = PHI(3);

Ro = [cos(psi)*cos(theta) cos(psi)*sin(theta)*sin(phi)-sin(psi)*cos(phi) cos(psi)*sin(theta)*cos(phi)+sin(psi)*sin(phi);
    sin(psi)*cos(theta) sin(psi)*sin(theta)*sin(phi)+cos(psi)*cos(phi) sin(psi)*sin(theta)*cos(phi)-cos(psi)*sin(phi);
    -sin(theta) cos(theta)*sin(phi) cos(theta)*cos(phi)];

Rel_Pos_local1 = Ro' * (r1 - ro);
Rel_Pos_local2 = Ro' * (r2 - ro);
Rel_Pos_local3 = Ro' * (r3 - ro);
Rel_Pos_local4 = Ro' * (r4 - ro);

end

== matlab function Simple_4Quad_payload_05/Dynamic model of the entire system/Drone absolute position computation ==
  data: q1 input; r1 output; r2 output; r3 output; r4 output; q2 input; q3 input; q4 input; d1 parameter; d2 parameter; l parameter; ro input; PHI input
function [r1,r2,r3,r4] = fcn(q1,q2,q3,q4,d1, d2, l,ro,PHI)

rho1 = [d1;0;0];
rho2 = [-d1;0;0];
rho3 = [0;d2;0];
rho4 = [0;-d2;0];

phi = PHI(1);
theta = PHI(2);
psi = PHI(3);

Ro = [cos(psi)*cos(theta) cos(psi)*sin(theta)*sin(phi)-sin(psi)*cos(phi) cos(psi)*sin(theta)*cos(phi)+sin(psi)*sin(phi);
    sin(psi)*cos(theta) sin(psi)*sin(theta)*sin(phi)+cos(psi)*cos(phi) sin(psi)*sin(theta)*cos(phi)-cos(psi)*sin(phi);
    -sin(theta) cos(theta)*sin(phi) cos(theta)*cos(phi)];

r1 = ro + Ro*rho1 + l*Ro*q1;
r2 = ro + Ro*rho2 + l*Ro*q2;
r3 = ro + Ro*rho3 + l*Ro*q3;
r4 = ro + Ro*rho4 + l*Ro*q4;

end

== matlab function Simple_4Quad_payload_05/Relative measurements/Relative acceleration measurements in payload local frame ==
  data: PHI input; Rel_Acc_local1 output; DDro input; DDr1 input; DDr2 input; DDr3 input; DDr4 input; Rel_Acc_local2 output; Rel_Acc_local3 output; Rel_Acc_local4 output
function [Rel_Acc_local1,Rel_Acc_local2,Rel_Acc_local3,Rel_Acc_local4] = fcn(PHI,DDro,DDr1,DDr2,DDr3,DDr4)

phi = PHI(1);
theta = PHI(2);
psi = PHI(3);

Ro = [cos(psi)*cos(theta) cos(psi)*sin(theta)*sin(phi)-sin(psi)*cos(phi) cos(psi)*sin(theta)*cos(phi)+sin(psi)*sin(phi);
    sin(psi)*cos(theta) sin(psi)*sin(theta)*sin(phi)+cos(psi)*cos(phi) sin(psi)*sin(theta)*cos(phi)-cos(psi)*sin(phi);
    -sin(theta) cos(theta)*sin(phi) cos(theta)*cos(phi)];

Rel_Acc_local1 = Ro' * (DDr1 - DDro);
Rel_Acc_local2 = Ro' * (DDr2 - DDro);
Rel_Acc_local3 = Ro' * (DDr3 - DDro);
Rel_Acc_local4 = Ro' * (DDr4 - DDro);

end

== matlab function Simple_4Quad_payload_05/Dynamic model of the entire system/Drone absolute acceleration computation ==
  data: q1 input; DDr1 output; DDr2 output; DDr3 output; DDr4 output; q2 input; q3 input; q4 input; Dq1 input; Dq2 input; Dq3 input; Dq4 input; DDq1 input; DDq2 input; DDq3 input; DDq4 input; All_rho parameter; l parameter; DDro input; PHI input; wo input; Dwo input
function [DDr1,DDr2,DDr3,DDr4] = fcn(q1,q2,q3,q4,Dq1,Dq2,Dq3,Dq4,DDq1,DDq2,DDq3,DDq4,All_rho, l,DDro,PHI,wo,Dwo)

rho1 = All_rho(1,:)';
rho2 = All_rho(2,:)';
rho3 = All_rho(3,:)';
rho4 = All_rho(4,:)';

phi = PHI(1);
theta = PHI(2);
psi = PHI(3);

wo_skew = [...
    0 -wo(3) wo(2);
    wo(3) 0 -wo(1);
    -wo(2) wo(1) 0];

Dwo_skew = [...
    0 -Dwo(3) Dwo(2);
    Dwo(3) 0 -Dwo(1);
    -Dwo(2) Dwo(1) 0];

Ro = [cos(psi)*cos(theta) cos(psi)*sin(theta)*sin(phi)-sin(psi)*cos(phi) cos(psi)*sin(theta)*cos(phi)+sin(psi)*sin(phi);
    sin(psi)*cos(theta) sin(psi)*sin(theta)*sin(phi)+cos(psi)*cos(phi) sin(psi)*sin(theta)*cos(phi)-cos(psi)*sin(phi);
    -sin(theta) cos(theta)*sin(phi) cos(theta)*cos(phi)];

DDr1 = DDro + Ro*wo_skew*wo_skew*rho1 + Ro*Dwo_skew*rho1 + l*Ro*wo_skew*wo_skew*q1 + l*Ro*Dwo_skew*q1 + 2*l*Ro*wo_skew*Dq1 + l*Ro*DDq1;
DDr2 = DDro + Ro*wo_skew*wo_skew*rho2 + Ro*Dwo_skew*rho2 + l*Ro*wo_skew*wo_skew*q2 + l*Ro*Dwo_skew*q2 + 2*l*Ro*wo_skew*Dq2 + l*Ro*DDq2;
DDr3 = DDro + Ro*wo_skew*wo_skew*rho3 + Ro*Dwo_skew*rho3 + l*Ro*wo_skew*wo_skew*q3 + l*Ro*Dwo_skew*q3 + 2*l*Ro*wo_skew*Dq3 + l*Ro*DDq3;
DDr4 = DDro + Ro*wo_skew*wo_skew*rho4 + Ro*Dwo_skew*rho4 + l*Ro*wo_skew*wo_skew*q4 + l*Ro*Dwo_skew*q4 + 2*l*Ro*wo_skew*Dq4 + l*Ro*DDq4;


end

== matlab function Simple_4Quad_payload_05/Controllers and Observers/Cotnroller and Observer - Agent1 /Rotational #1/output definition ==
  data: u input; ur output
function ur = fcn(u)

ur = u(4:6);

end

== matlab function Simple_4Quad_payload_05/Controllers and Observers/Controller and Observer - Agent2/Rotational #2/output definition ==
  data: u input; ur output
function ur = fcn(u)

ur = u(4:6);

end

== matlab function Simple_4Quad_payload_05/Controllers and Observers/Cotnroller and Observer - Agent1 /Rotational #1/CARE ==
  data: P input; a_hat input; BR parameter; R parameter; DP output; QR parameter
function DP = fcn(P,a_hat,BR,R,QR)

DP = a_hat*P + P*a_hat' - P*BR*R*BR'*P + 2*QR;

end

== matlab function Simple_4Quad_payload_05/Controllers and Observers/Controlelr and Observer - Agent3/Rotational #3/output definition ==
  data: u input; ur output
function ur = fcn(u)

ur = u(4:6);

end

== matlab function Simple_4Quad_payload_05/Controllers and Observers/Controller and Observer - Agent4/Rotational #4/output definition ==
  data: u input; ur output
function ur = fcn(u)

ur = u(4:6);

end

== matlab function Simple_4Quad_payload_05/Controllers and Observers/Cotnroller and Observer - Agent1 /Rotational #1/Differentiator/Sliding differentiator ==
  data: u output; u1 input; e input; n parameter; k1 parameter
function u = fcn(u1,e,n,k1)

b=k1;

ABS = zeros(n,1);
for i=1:n
    if e(i)>0
        ABS(i) = e(i);
    else
        ABS(i) = -e(i);
    end
end
SGN = e ./ (ABS + 0.01);

u = u1 - b*(ABS.^0.5).*SGN;

end

== matlab function Simple_4Quad_payload_05/Controllers and Observers/Cotnroller and Observer - Agent1 /Controller Interpreter #1 ==
  data: ut_1 input; PHI_d_1 output
function PHI_d_1 = fcn(ut_1)

%%
fT_1 = sqrt((ut_1(1)^2)+(ut_1(2)^2)+(ut_1(3)^2));
psi_d_1 = 0;
phi_d_1 = asin( min(max(((sin(psi_d_1)*ut_1(1) - cos(psi_d_1)*ut_1(2)) / (fT_1+1e-3)),-1),1) );
theta_d_1 = atan( (cos(psi_d_1)*ut_1(1) + sin(psi_d_1)*ut_1(2)) / (ut_1(3)+1e-3) );
PHI_d_1 = [phi_d_1;theta_d_1;psi_d_1]; 

end

== matlab function Simple_4Quad_payload_05/Controllers and Observers/Cotnroller and Observer - Agent1 /Rotational #1/Differentiator/Sliding differentiator1 ==
  data: Du1 output; e input; n parameter; k2 parameter
function Du1 = fcn(e,n,k2)

a=k2;

ABS = zeros(n,1);
for i=1:n
    if e(i)>0
        ABS(i) = e(i);
    else
        ABS(i) = -e(i);
    end
end
SGN = e ./ (ABS + 0.01);

Du1 = - a*SGN;

end

== matlab function Simple_4Quad_payload_05/Controllers and Observers/Cotnroller and Observer - Agent1 /Rotational #1/g-Estimator ==
  data: sigma input; g_hat input; P input; rho_1 parameter; gamma_1 parameter; Dg_hat output
function Dg_hat = fcn(sigma,g_hat,P,rho_1,gamma_1)

Dg_hat = - gamma_1 * P * sigma - rho_1 * gamma_1 * g_hat;

end

== matlab function Simple_4Quad_payload_05/Controllers and Observers/Cotnroller and Observer - Agent1 /Rotational #1/g-Estimator1 ==
  data: sigma input; x input; P input; rho_0 parameter; gamma_0 parameter; Da_hat output; a_hat input
function Da_hat = fcn(sigma,x,P,rho_0,gamma_0,a_hat)

DVa_hat = - gamma_0 * P * diag(sigma) * (x - sigma) - rho_0 * gamma_0 * diag(a_hat);

Da_hat = diag(DVa_hat);

end

== matlab function Simple_4Quad_payload_05/Controllers and Observers/Cotnroller and Observer - Agent1 /Rotational #1/main ==
  data: sigma input; zeta input; u output; Dy_d input; R parameter; P input; a_hat input; BR parameter; g_hat input; x input; QR parameter; BBT_inv parameter; n parameter
function u = fcn(sigma,zeta,Dy_d,R,P,a_hat,BR,g_hat,x,QR,BBT_inv,n)

u1 = (1/2) * R * BR' * P * sigma;
u2 = BBT_inv * (Dy_d - a_hat*x + (eye(n) + 2*(((P)^(-1)*QR)) + a_hat)*sigma - g_hat - zeta) - (3/4) * R * BR' * P * sigma;

u = u1 + u2;

end

== matlab function Simple_4Quad_payload_05/Controllers and Observers/Cotnroller and Observer - Agent1 /Rotational #1/variable change ==
  data: X input; Xd input; x_mod output; u input; xd_mod output; e_mod output
function [x_mod,xd_mod,e_mod] = fcn(X,Xd,u)

x_mod = X;

xd_mod = [Xd;u(1:3)];

e_mod = xd_mod - x_mod;


end

== matlab function Simple_4Quad_payload_05/Rotational Controller Log/For matrix Plot/MATLAB Function ==
  data: u input; y output
function y = fcn(u)
S1 = size(u,1);
S2 = size(u,2);

y = zeros(S1*S2,1);
num = 0;
for i=1:S1
    for j=1:S2
        num = num + 1;
        y(num,1) = u(i,j);
    end
end

end

== matlab function Simple_4Quad_payload_05/Rotational Controller Log/For matrix Plot1/MATLAB Function ==
  data: u input; y output
function y = fcn(u)
S1 = size(u,1);
S2 = size(u,2);

y = zeros(S1*S2,1);
num = 0;
for i=1:S1
    for j=1:S2
        num = num + 1;
        y(num,1) = u(i,j);
    end
end

end

== matlab function Simple_4Quad_payload_05/Rotational Controller Log/For matrix Plot2/MATLAB Function ==
  data: u input; y output
function y = fcn(u)
S1 = size(u,1);
S2 = size(u,2);

y = zeros(S1*S2,1);
num = 0;
for i=1:S1
    for j=1:S2
        num = num + 1;
        y(num,1) = u(i,j);
    end
end

end

== matlab function Simple_4Quad_payload_05/Rotational Controller Log/For matrix Plot3/MATLAB Function ==
  data: u input; y output
function y = fcn(u)
S1 = size(u,1);
S2 = size(u,2);

y = zeros(S1*S2,1);
num = 0;
for i=1:S1
    for j=1:S2
        num = num + 1;
        y(num,1) = u(i,j);
    end
end

end

== matlab function Simple_4Quad_payload_05/Rotational Controller Log/For matrix Plot4/MATLAB Function ==
  data: u input; y output
function y = fcn(u)
S1 = size(u,1);
S2 = size(u,2);

y = zeros(S1*S2,1);
num = 0;
for i=1:S1
    for j=1:S2
        num = num + 1;
        y(num,1) = u(i,j);
    end
end

end

== matlab function Simple_4Quad_payload_05/Rotational Controller Log/For matrix Plot5/MATLAB Function ==
  data: u input; y output
function y = fcn(u)
S1 = size(u,1);
S2 = size(u,2);

y = zeros(S1*S2,1);
num = 0;
for i=1:S1
    for j=1:S2
        num = num + 1;
        y(num,1) = u(i,j);
    end
end

end

== matlab function Simple_4Quad_payload_05/Rotational Controller Log/For matrix Plot6/MATLAB Function ==
  data: u input; y output
function y = fcn(u)
S1 = size(u,1);
S2 = size(u,2);

y = zeros(S1*S2,1);
num = 0;
for i=1:S1
    for j=1:S2
        num = num + 1;
        y(num,1) = u(i,j);
    end
end

end

== matlab function Simple_4Quad_payload_05/Rotational Controller Log/For matrix Plot7/MATLAB Function ==
  data: u input; y output
function y = fcn(u)
S1 = size(u,1);
S2 = size(u,2);

y = zeros(S1*S2,1);
num = 0;
for i=1:S1
    for j=1:S2
        num = num + 1;
        y(num,1) = u(i,j);
    end
end

end
